simulink model "HANcoder_E407_DYS_MP"  (R2018b)
settings: Solver=FixedStepDiscrete  StartTime=0.0  StopTime=1  FixedStep=0.01  RelTol=1e-3
PreLoadFcn:
  | librarySetup
  | eval([bdroot,'_startup']) %Calling [modelName]_startup.m
values from neighbouring files (symbols this model uses):
  basic_cycle_duration_bc0 = TM_Reset_Board   + COMP_duration    (= 212)    [HANcoder_E407_DYS_MP_startup.m]
  basic_cycle_duration_bc1 = basic_cycle_duration_bc0    (= 212)    [HANcoder_E407_DYS_MP_startup.m]
  comm_delay_estimation1 = round(comm_delay_measured1*hardware_granularity/frequency_IRQ)    [HANcoder_E407_DYS_MP_startup.m]
  comm_delay_estimation2 = round(comm_delay_measured2*hardware_granularity/frequency_IRQ)    [HANcoder_E407_DYS_MP_startup.m]
  COMM_Phase1 = Simulink.Parameter    [HANcoder_E407_DYS_MP_startup.m]
  COMM_Phase2 = Simulink.Parameter    [HANcoder_E407_DYS_MP_startup.m]
  frequency_IRQ = 500    [HANcoder_E407_DYS_MP_startup.m]
  HantuneAngleSp = Simulink.Parameter    [HANcoder_E407_DYS_MP_startup.m]
  idle_time_init = basic_cycle_duration_bc0 + basic_cycle_duration_bc1    (= 424)    [HANcoder_E407_DYS_MP_startup.m]
  matrix_rows = 2    [HANcoder_E407_DYS_MP_startup.m]
  positionD = Simulink.Parameter    [HANcoder_E407_DYS_MP_startup.m]
  positionI = Simulink.Parameter    [HANcoder_E407_DYS_MP_startup.m]
  positionP = Simulink.Parameter    [HANcoder_E407_DYS_MP_startup.m]
undefined symbols (not defined in the file or in its folder): A1, CON2, CON4, D13, Dposition, Iposition, Pposition
libraries: HANcoder_STM32_Target x33, dspswit3 x16, simulink x2, simulink_extras x2, dspstat3 x1
(part 7 of 10)

== system HANcoder_E407_DYS_MP/HANcoder STM32 Target - E407-STM32 algorithm/4.TTA Can System/4.3 TTA System/4.3.3 Matrix Cycle Manager/4.3.3.1 Controller Matrix Cycle Truck Boards 1 2 and 3/4.3.3.1.2 controller basic cycle 0.2/Receive Truck 1 Board 1 Calc Steering Angle/Receive can message ==
  Can_ID : Inport
  Enable : EnablePort  ShowOutputPort=on
  CAN receive : Subsystem  Tag=HANcoder_TARGET_STM32_E407  AncestorBlock=HANcoder_STM32_Target/STM32-E407/CAN/CAN/CAN receive  mask(CAN receive){canBus=CAN 1, outputNumber=1, dataType=uint8, byteOrder=off, tsamp=-1}
      mask prompts: canBus "CAN channel"; outputNumber "Output ports"; dataType "Output datatype"; byteOrder "Byte order: Checked = MSB first, unchecked = LSB first."; tsamp "Sample time"
      mask help:
      | Function
      | ==========
      | Receive the newest message from the specified CAN channel.
      |
      | Parameters
      | ==========
      | CAN channel:             The CAN channel to send the message on.
      | Output ports:             The amount of output ports
      | Output datatype:       The datatype of the output ports
      | Byte order:                 Select MSB or LSB first
      | Sample time:              -1 or divisible by base sample time [seconds]
      |
      | Input
      | ==========
      | Port 1:                       CAN ID(uint32) in hexadecimal ie: hex2dec('0a')
      |
      | Output
      | ==========
      | Port 1:                       Checks for new message(int8)
      | Port 2..9                     Message data
      mask init:
      | sfcn_can_receive_mcb(canBus, outputNumber, dataType, byteOrder)
      settings: MoveFcn=drawLogos
      mask Help: web('sfcn_can_receive.html');
      mask TypeOptions canBus: CAN 1 | CAN 2
      mask TypeOptions dataType: int8 | uint8 | int16 | uint16 | int32 | uint32 | boolean
      mask Display:
      | fprintf('Receive on\nCAN %x', canBus);
      | port_label('output', 1, 'new');
      | port_label('input', 1, 'ID');patch([75 81 81],[8 14 2],[1 0 0]);patch([83 83 89],[14 2 8],[0 0 0.35]);
  CAN receive2 : Subsystem  Tag=HANcoder_TARGET_STM32_E407  AncestorBlock=HANcoder_STM32_Target/STM32-E407/CAN/CAN/CAN receive  mask(CAN receive){canBus=CAN 2, outputNumber=1, dataType=uint8, byteOrder=off, tsamp=-1}
      mask prompts: canBus "CAN channel"; outputNumber "Output ports"; dataType "Output datatype"; byteOrder "Byte order: Checked = MSB first, unchecked = LSB first."; tsamp "Sample time"
      mask help:
      | Function
      | ==========
      | Receive the newest message from the specified CAN channel.
      |
      | Parameters
      | ==========
      | CAN channel:             The CAN channel to send the message on.
      | Output ports:             The amount of output ports
      | Output datatype:       The datatype of the output ports
      | Byte order:                 Select MSB or LSB first
      | Sample time:              -1 or divisible by base sample time [seconds]
      |
      | Input
      | ==========
      | Port 1:                       CAN ID(uint32) in hexadecimal ie: hex2dec('0a')
      |
      | Output
      | ==========
      | Port 1:                       Checks for new message(int8)
      | Port 2..9                     Message data
      mask init:
      | sfcn_can_receive_mcb(canBus, outputNumber, dataType, byteOrder)
      settings: MoveFcn=drawLogos
      mask Help: web('sfcn_can_receive.html');
      mask TypeOptions canBus: CAN 1 | CAN 2
      mask TypeOptions dataType: int8 | uint8 | int16 | uint16 | int32 | uint32 | boolean
      mask Display:
      | fprintf('Receive on\nCAN %x', canBus);
      | port_label('output', 1, 'new');
      | port_label('input', 1, 'ID');patch([75 81 81],[8 14 2],[1 0 0]);patch([83 83 89],[14 2 8],[0 0 0.35]);
  Can1Port1 : Outport
  Can1Receive : Outport  Port=2
  Can2Port2 : Outport  Port=3
  Can2Receive : Outport  Port=4
  wires:
  CAN receive/2(Out2) -> Can1Port1/1
  CAN receive/1(Out1) -> Can1Receive/1
  Can_ID/1 -> CAN receive2/1(In1), CAN receive/1(In1)
  CAN receive2/1(Out1) -> Can2Receive/1
  CAN receive2/2(Out2) -> Can2Port2/1

== system HANcoder_E407_DYS_MP/HANcoder STM32 Target - E407-STM32 algorithm/4.TTA Can System/4.3 TTA System/4.3.3 Matrix Cycle Manager/4.3.3.1 Controller Matrix Cycle Truck Boards 1 2 and 3/4.3.3.1.2 controller basic cycle 0.2/Receive Truck 1 Board 1 Calc Steering Angle1/Desync calculation ==
  New_msg_CAN1 : Inport
  Can1_Msg : Inport  Port=2
  Can2_Msg : Inport  Port=3
  Enable : EnablePort  ShowOutputPort=on
  Switch1 : Switch  Priority=22  Criteria=u2 > Threshold
  Vote : Outport
  wires:
  New_msg_CAN1/1 -> Switch1/2
  Can1_Msg/1 -> Switch1/1
  Can2_Msg/1 -> Switch1/3
  Switch1/1 -> Vote/1

== system HANcoder_E407_DYS_MP/HANcoder STM32 Target - E407-STM32 algorithm/4.TTA Can System/4.3 TTA System/4.3.3 Matrix Cycle Manager/4.3.3.1 Controller Matrix Cycle Truck Boards 1 2 and 3/4.3.3.1.2 controller basic cycle 0.2/Receive Truck 1 Board 1 Calc Steering Angle1/Receive can message ==
  Can_ID : Inport
  Enable : EnablePort  ShowOutputPort=on
  CAN receive : Subsystem  Tag=HANcoder_TARGET_STM32_E407  AncestorBlock=HANcoder_STM32_Target/STM32-E407/CAN/CAN/CAN receive  mask(CAN receive){canBus=CAN 1, outputNumber=1, dataType=uint8, byteOrder=off, tsamp=-1}
      mask prompts: canBus "CAN channel"; outputNumber "Output ports"; dataType "Output datatype"; byteOrder "Byte order: Checked = MSB first, unchecked = LSB first."; tsamp "Sample time"
      mask help:
      | Function
      | ==========
      | Receive the newest message from the specified CAN channel.
      |
      | Parameters
      | ==========
      | CAN channel:             The CAN channel to send the message on.
      | Output ports:             The amount of output ports
      | Output datatype:       The datatype of the output ports
      | Byte order:                 Select MSB or LSB first
      | Sample time:              -1 or divisible by base sample time [seconds]
      |
      | Input
      | ==========
      | Port 1:                       CAN ID(uint32) in hexadecimal ie: hex2dec('0a')
      |
      | Output
      | ==========
      | Port 1:                       Checks for new message(int8)
      | Port 2..9                     Message data
      mask init:
      | sfcn_can_receive_mcb(canBus, outputNumber, dataType, byteOrder)
      settings: MoveFcn=drawLogos
      mask Help: web('sfcn_can_receive.html');
      mask TypeOptions canBus: CAN 1 | CAN 2
      mask TypeOptions dataType: int8 | uint8 | int16 | uint16 | int32 | uint32 | boolean
      mask Display:
      | fprintf('Receive on\nCAN %x', canBus);
      | port_label('output', 1, 'new');
      | port_label('input', 1, 'ID');patch([75 81 81],[8 14 2],[1 0 0]);patch([83 83 89],[14 2 8],[0 0 0.35]);
  CAN receive2 : Subsystem  Tag=HANcoder_TARGET_STM32_E407  AncestorBlock=HANcoder_STM32_Target/STM32-E407/CAN/CAN/CAN receive  mask(CAN receive){canBus=CAN 2, outputNumber=1, dataType=uint8, byteOrder=off, tsamp=-1}
      mask prompts: canBus "CAN channel"; outputNumber "Output ports"; dataType "Output datatype"; byteOrder "Byte order: Checked = MSB first, unchecked = LSB first."; tsamp "Sample time"
      mask help:
      | Function
      | ==========
      | Receive the newest message from the specified CAN channel.
      |
      | Parameters
      | ==========
      | CAN channel:             The CAN channel to send the message on.
      | Output ports:             The amount of output ports
      | Output datatype:       The datatype of the output ports
      | Byte order:                 Select MSB or LSB first
      | Sample time:              -1 or divisible by base sample time [seconds]
      |
      | Input
      | ==========
      | Port 1:                       CAN ID(uint32) in hexadecimal ie: hex2dec('0a')
      |
      | Output
      | ==========
      | Port 1:                       Checks for new message(int8)
      | Port 2..9                     Message data
      mask init:
      | sfcn_can_receive_mcb(canBus, outputNumber, dataType, byteOrder)
      settings: MoveFcn=drawLogos
      mask Help: web('sfcn_can_receive.html');
      mask TypeOptions canBus: CAN 1 | CAN 2
      mask TypeOptions dataType: int8 | uint8 | int16 | uint16 | int32 | uint32 | boolean
      mask Display:
      | fprintf('Receive on\nCAN %x', canBus);
      | port_label('output', 1, 'new');
      | port_label('input', 1, 'ID');patch([75 81 81],[8 14 2],[1 0 0]);patch([83 83 89],[14 2 8],[0 0 0.35]);
  Can1Port1 : Outport
  Can1Receive : Outport  Port=2
  Can2Port2 : Outport  Port=3
  Can2Receive : Outport  Port=4
  wires:
  CAN receive/2(Out2) -> Can1Port1/1
  CAN receive/1(Out1) -> Can1Receive/1
  Can_ID/1 -> CAN receive2/1(In1), CAN receive/1(In1)
  CAN receive2/1(Out1) -> Can2Receive/1
  CAN receive2/2(Out2) -> Can2Port2/1

== system HANcoder_E407_DYS_MP/HANcoder STM32 Target - E407-STM32 algorithm/4.TTA Can System/4.3 TTA System/4.3.3 Matrix Cycle Manager/4.3.3.1 Controller Matrix Cycle Truck Boards 1 2 and 3/4.3.3.1.2 controller basic cycle 0.2/Receive Truck 1 Board 1 Calc Steering Angle2/Desync calculation ==
  New_msg_CAN1 : Inport
  Can1_Msg : Inport  Port=2
  Can2_Msg : Inport  Port=3
  Enable : EnablePort  ShowOutputPort=on
  Switch1 : Switch  Priority=22  Criteria=u2 > Threshold
  Vote : Outport
  wires:
  New_msg_CAN1/1 -> Switch1/2
  Can1_Msg/1 -> Switch1/1
  Can2_Msg/1 -> Switch1/3
  Switch1/1 -> Vote/1

== system HANcoder_E407_DYS_MP/HANcoder STM32 Target - E407-STM32 algorithm/4.TTA Can System/4.3 TTA System/4.3.3 Matrix Cycle Manager/4.3.3.1 Controller Matrix Cycle Truck Boards 1 2 and 3/4.3.3.1.2 controller basic cycle 0.2/Receive Truck 1 Board 1 Calc Steering Angle2/Receive can message ==
  Can_ID : Inport
  Enable : EnablePort  ShowOutputPort=on
  CAN receive : Subsystem  Tag=HANcoder_TARGET_STM32_E407  AncestorBlock=HANcoder_STM32_Target/STM32-E407/CAN/CAN/CAN receive  mask(CAN receive){canBus=CAN 1, outputNumber=1, dataType=uint8, byteOrder=off, tsamp=-1}
      mask prompts: canBus "CAN channel"; outputNumber "Output ports"; dataType "Output datatype"; byteOrder "Byte order: Checked = MSB first, unchecked = LSB first."; tsamp "Sample time"
      mask help:
      | Function
      | ==========
      | Receive the newest message from the specified CAN channel.
      |
      | Parameters
      | ==========
      | CAN channel:             The CAN channel to send the message on.
      | Output ports:             The amount of output ports
      | Output datatype:       The datatype of the output ports
      | Byte order:                 Select MSB or LSB first
      | Sample time:              -1 or divisible by base sample time [seconds]
      |
      | Input
      | ==========
      | Port 1:                       CAN ID(uint32) in hexadecimal ie: hex2dec('0a')
      |
      | Output
      | ==========
      | Port 1:                       Checks for new message(int8)
      | Port 2..9                     Message data
      mask init:
      | sfcn_can_receive_mcb(canBus, outputNumber, dataType, byteOrder)
      settings: MoveFcn=drawLogos
      mask Help: web('sfcn_can_receive.html');
      mask TypeOptions canBus: CAN 1 | CAN 2
      mask TypeOptions dataType: int8 | uint8 | int16 | uint16 | int32 | uint32 | boolean
      mask Display:
      | fprintf('Receive on\nCAN %x', canBus);
      | port_label('output', 1, 'new');
      | port_label('input', 1, 'ID');patch([75 81 81],[8 14 2],[1 0 0]);patch([83 83 89],[14 2 8],[0 0 0.35]);
  CAN receive2 : Subsystem  Tag=HANcoder_TARGET_STM32_E407  AncestorBlock=HANcoder_STM32_Target/STM32-E407/CAN/CAN/CAN receive  mask(CAN receive){canBus=CAN 2, outputNumber=1, dataType=uint8, byteOrder=off, tsamp=-1}
      mask prompts: canBus "CAN channel"; outputNumber "Output ports"; dataType "Output datatype"; byteOrder "Byte order: Checked = MSB first, unchecked = LSB first."; tsamp "Sample time"
      mask help:
      | Function
      | ==========
      | Receive the newest message from the specified CAN channel.
      |
      | Parameters
      | ==========
      | CAN channel:             The CAN channel to send the message on.
      | Output ports:             The amount of output ports
      | Output datatype:       The datatype of the output ports
      | Byte order:                 Select MSB or LSB first
      | Sample time:              -1 or divisible by base sample time [seconds]
      |
      | Input
      | ==========
      | Port 1:                       CAN ID(uint32) in hexadecimal ie: hex2dec('0a')
      |
      | Output
      | ==========
      | Port 1:                       Checks for new message(int8)
      | Port 2..9                     Message data
      mask init:
      | sfcn_can_receive_mcb(canBus, outputNumber, dataType, byteOrder)
      settings: MoveFcn=drawLogos
      mask Help: web('sfcn_can_receive.html');
      mask TypeOptions canBus: CAN 1 | CAN 2
      mask TypeOptions dataType: int8 | uint8 | int16 | uint16 | int32 | uint32 | boolean
      mask Display:
      | fprintf('Receive on\nCAN %x', canBus);
      | port_label('output', 1, 'new');
      | port_label('input', 1, 'ID');patch([75 81 81],[8 14 2],[1 0 0]);patch([83 83 89],[14 2 8],[0 0 0.35]);
  Can1Port1 : Outport
  Can1Receive : Outport  Port=2
  Can2Port2 : Outport  Port=3
  Can2Receive : Outport  Port=4
  wires:
  CAN receive/2(Out2) -> Can1Port1/1
  CAN receive/1(Out1) -> Can1Receive/1
  Can_ID/1 -> CAN receive2/1(In1), CAN receive/1(In1)
  CAN receive2/1(Out1) -> Can2Receive/1
  CAN receive2/2(Out2) -> Can2Port2/1

== system HANcoder_E407_DYS_MP/HANcoder STM32 Target - E407-STM32 algorithm/4.TTA Can System/4.3 TTA System/4.3.3 Matrix Cycle Manager/4.3.3.1 Controller Matrix Cycle Truck Boards 1 2 and 3/4.3.3.1.2 controller basic cycle 0.2/Receive Truck 1 Board 1 Calc Steering Angle3/Desync calculation ==
  New_msg_CAN1 : Inport
  Can1_Msg : Inport  Port=2
  Can2_Msg : Inport  Port=3
  Enable : EnablePort  ShowOutputPort=on
  Switch1 : Switch  Priority=22  Criteria=u2 > Threshold
  Vote : Outport
  wires:
  New_msg_CAN1/1 -> Switch1/2
  Can1_Msg/1 -> Switch1/1
  Can2_Msg/1 -> Switch1/3
  Switch1/1 -> Vote/1

== system HANcoder_E407_DYS_MP/HANcoder STM32 Target - E407-STM32 algorithm/4.TTA Can System/4.3 TTA System/4.3.3 Matrix Cycle Manager/4.3.3.1 Controller Matrix Cycle Truck Boards 1 2 and 3/4.3.3.1.2 controller basic cycle 0.2/Receive Truck 1 Board 1 Calc Steering Angle3/Receive can message ==
  Can_ID : Inport
  Enable : EnablePort  ShowOutputPort=on
  CAN receive : Subsystem  Tag=HANcoder_TARGET_STM32_E407  AncestorBlock=HANcoder_STM32_Target/STM32-E407/CAN/CAN/CAN receive  mask(CAN receive){canBus=CAN 1, outputNumber=1, dataType=uint8, byteOrder=off, tsamp=-1}
      mask prompts: canBus "CAN channel"; outputNumber "Output ports"; dataType "Output datatype"; byteOrder "Byte order: Checked = MSB first, unchecked = LSB first."; tsamp "Sample time"
      mask help:
      | Function
      | ==========
      | Receive the newest message from the specified CAN channel.
      |
      | Parameters
      | ==========
      | CAN channel:             The CAN channel to send the message on.
      | Output ports:             The amount of output ports
      | Output datatype:       The datatype of the output ports
      | Byte order:                 Select MSB or LSB first
      | Sample time:              -1 or divisible by base sample time [seconds]
      |
      | Input
      | ==========
      | Port 1:                       CAN ID(uint32) in hexadecimal ie: hex2dec('0a')
      |
      | Output
      | ==========
      | Port 1:                       Checks for new message(int8)
      | Port 2..9                     Message data
      mask init:
      | sfcn_can_receive_mcb(canBus, outputNumber, dataType, byteOrder)
      settings: MoveFcn=drawLogos
      mask Help: web('sfcn_can_receive.html');
      mask TypeOptions canBus: CAN 1 | CAN 2
      mask TypeOptions dataType: int8 | uint8 | int16 | uint16 | int32 | uint32 | boolean
      mask Display:
      | fprintf('Receive on\nCAN %x', canBus);
      | port_label('output', 1, 'new');
      | port_label('input', 1, 'ID');patch([75 81 81],[8 14 2],[1 0 0]);patch([83 83 89],[14 2 8],[0 0 0.35]);
  CAN receive2 : Subsystem  Tag=HANcoder_TARGET_STM32_E407  AncestorBlock=HANcoder_STM32_Target/STM32-E407/CAN/CAN/CAN receive  mask(CAN receive){canBus=CAN 2, outputNumber=1, dataType=uint8, byteOrder=off, tsamp=-1}
      mask prompts: canBus "CAN channel"; outputNumber "Output ports"; dataType "Output datatype"; byteOrder "Byte order: Checked = MSB first, unchecked = LSB first."; tsamp "Sample time"
      mask help:
      | Function
      | ==========
      | Receive the newest message from the specified CAN channel.
      |
      | Parameters
      | ==========
      | CAN channel:             The CAN channel to send the message on.
      | Output ports:             The amount of output ports
      | Output datatype:       The datatype of the output ports
      | Byte order:                 Select MSB or LSB first
      | Sample time:              -1 or divisible by base sample time [seconds]
      |
      | Input
      | ==========
      | Port 1:                       CAN ID(uint32) in hexadecimal ie: hex2dec('0a')
      |
      | Output
      | ==========
      | Port 1:                       Checks for new message(int8)
      | Port 2..9                     Message data
      mask init:
      | sfcn_can_receive_mcb(canBus, outputNumber, dataType, byteOrder)
      settings: MoveFcn=drawLogos
      mask Help: web('sfcn_can_receive.html');
      mask TypeOptions canBus: CAN 1 | CAN 2
      mask TypeOptions dataType: int8 | uint8 | int16 | uint16 | int32 | uint32 | boolean
      mask Display:
      | fprintf('Receive on\nCAN %x', canBus);
      | port_label('output', 1, 'new');
      | port_label('input', 1, 'ID');patch([75 81 81],[8 14 2],[1 0 0]);patch([83 83 89],[14 2 8],[0 0 0.35]);
  Can1Port1 : Outport
  Can1Receive : Outport  Port=2
  Can2Port2 : Outport  Port=3
  Can2Receive : Outport  Port=4
  wires:
  CAN receive/2(Out2) -> Can1Port1/1
  CAN receive/1(Out1) -> Can1Receive/1
  Can_ID/1 -> CAN receive2/1(In1), CAN receive/1(In1)
  CAN receive2/1(Out1) -> Can2Receive/1
  CAN receive2/2(Out2) -> Can2Port2/1

== system HANcoder_E407_DYS_MP/HANcoder STM32 Target - E407-STM32 algorithm/4.TTA Can System/4.3 TTA System/4.3.3 Matrix Cycle Manager/4.3.3.1 Controller Matrix Cycle Truck Boards 1 2 and 3/4.3.3.1.2 controller basic cycle 0.2/Receive Truck 2 Board 2 Calc Steering Angle/Desync calculation ==
  New_msg_CAN1 : Inport
  Can1_Msg : Inport  Port=2
  Can2_Msg : Inport  Port=3
  Enable : EnablePort  ShowOutputPort=on
  Switch1 : Switch  Priority=22  Criteria=u2 > Threshold
  Vote : Outport
  wires:
  New_msg_CAN1/1 -> Switch1/2
  Can1_Msg/1 -> Switch1/1
  Can2_Msg/1 -> Switch1/3
  Switch1/1 -> Vote/1

== system HANcoder_E407_DYS_MP/HANcoder STM32 Target - E407-STM32 algorithm/4.TTA Can System/4.3 TTA System/4.3.3 Matrix Cycle Manager/4.3.3.1 Controller Matrix Cycle Truck Boards 1 2 and 3/4.3.3.1.2 controller basic cycle 0.2/Receive Truck 2 Board 2 Calc Steering Angle/Receive can message ==
  Can_ID : Inport
  Enable : EnablePort  ShowOutputPort=on
  CAN receive : Subsystem  Tag=HANcoder_TARGET_STM32_E407  AncestorBlock=HANcoder_STM32_Target/STM32-E407/CAN/CAN/CAN receive  mask(CAN receive){canBus=CAN 1, outputNumber=1, dataType=uint8, byteOrder=off, tsamp=-1}
      mask prompts: canBus "CAN channel"; outputNumber "Output ports"; dataType "Output datatype"; byteOrder "Byte order: Checked = MSB first, unchecked = LSB first."; tsamp "Sample time"
      mask help:
      | Function
      | ==========
      | Receive the newest message from the specified CAN channel.
      |
      | Parameters
      | ==========
      | CAN channel:             The CAN channel to send the message on.
      | Output ports:             The amount of output ports
      | Output datatype:       The datatype of the output ports
      | Byte order:                 Select MSB or LSB first
      | Sample time:              -1 or divisible by base sample time [seconds]
      |
      | Input
      | ==========
      | Port 1:                       CAN ID(uint32) in hexadecimal ie: hex2dec('0a')
      |
      | Output
      | ==========
      | Port 1:                       Checks for new message(int8)
      | Port 2..9                     Message data
      mask init:
      | sfcn_can_receive_mcb(canBus, outputNumber, dataType, byteOrder)
      settings: MoveFcn=drawLogos
      mask Help: web('sfcn_can_receive.html');
      mask TypeOptions canBus: CAN 1 | CAN 2
      mask TypeOptions dataType: int8 | uint8 | int16 | uint16 | int32 | uint32 | boolean
      mask Display:
      | fprintf('Receive on\nCAN %x', canBus);
      | port_label('output', 1, 'new');
      | port_label('input', 1, 'ID');patch([75 81 81],[8 14 2],[1 0 0]);patch([83 83 89],[14 2 8],[0 0 0.35]);
  CAN receive2 : Subsystem  Tag=HANcoder_TARGET_STM32_E407  AncestorBlock=HANcoder_STM32_Target/STM32-E407/CAN/CAN/CAN receive  mask(CAN receive){canBus=CAN 2, outputNumber=1, dataType=uint8, byteOrder=off, tsamp=-1}
      mask prompts: canBus "CAN channel"; outputNumber "Output ports"; dataType "Output datatype"; byteOrder "Byte order: Checked = MSB first, unchecked = LSB first."; tsamp "Sample time"
      mask help:
      | Function
      | ==========
      | Receive the newest message from the specified CAN channel.
      |
      | Parameters
      | ==========
      | CAN channel:             The CAN channel to send the message on.
      | Output ports:             The amount of output ports
      | Output datatype:       The datatype of the output ports
      | Byte order:                 Select MSB or LSB first
      | Sample time:              -1 or divisible by base sample time [seconds]
      |
      | Input
      | ==========
      | Port 1:                       CAN ID(uint32) in hexadecimal ie: hex2dec('0a')
      |
      | Output
      | ==========
      | Port 1:                       Checks for new message(int8)
      | Port 2..9                     Message data
      mask init:
      | sfcn_can_receive_mcb(canBus, outputNumber, dataType, byteOrder)
      settings: MoveFcn=drawLogos
      mask Help: web('sfcn_can_receive.html');
      mask TypeOptions canBus: CAN 1 | CAN 2
      mask TypeOptions dataType: int8 | uint8 | int16 | uint16 | int32 | uint32 | boolean
      mask Display:
      | fprintf('Receive on\nCAN %x', canBus);
      | port_label('output', 1, 'new');
      | port_label('input', 1, 'ID');patch([75 81 81],[8 14 2],[1 0 0]);patch([83 83 89],[14 2 8],[0 0 0.35]);
  Can1Port1 : Outport
  Can1Receive : Outport  Port=2
  Can2Port2 : Outport  Port=3
  Can2Receive : Outport  Port=4
  wires:
  CAN receive/2(Out2) -> Can1Port1/1
  CAN receive/1(Out1) -> Can1Receive/1
  Can_ID/1 -> CAN receive2/1(In1), CAN receive/1(In1)
  CAN receive2/1(Out1) -> Can2Receive/1
  CAN receive2/2(Out2) -> Can2Port2/1

== system HANcoder_E407_DYS_MP/HANcoder STM32 Target - E407-STM32 algorithm/4.TTA Can System/4.3 TTA System/4.3.3 Matrix Cycle Manager/4.3.3.1 Controller Matrix Cycle Truck Boards 1 2 and 3/4.3.3.1.2 controller basic cycle 0.2/Receive Truck 3 Board 3 Calc Steering Angle/Desync calculation ==
  New_msg_CAN1 : Inport
  Can1_Msg : Inport  Port=2
  Can2_Msg : Inport  Port=3
  Enable : EnablePort  ShowOutputPort=on
  Switch1 : Switch  Priority=22  Criteria=u2 > Threshold
  Vote : Outport
  wires:
  New_msg_CAN1/1 -> Switch1/2
  Can1_Msg/1 -> Switch1/1
  Can2_Msg/1 -> Switch1/3
  Switch1/1 -> Vote/1

== system HANcoder_E407_DYS_MP/HANcoder STM32 Target - E407-STM32 algorithm/4.TTA Can System/4.3 TTA System/4.3.3 Matrix Cycle Manager/4.3.3.1 Controller Matrix Cycle Truck Boards 1 2 and 3/4.3.3.1.2 controller basic cycle 0.2/Receive Truck 3 Board 3 Calc Steering Angle/Receive can message ==
  Can_ID : Inport
  Enable : EnablePort  ShowOutputPort=on
  CAN receive : Subsystem  Tag=HANcoder_TARGET_STM32_E407  AncestorBlock=HANcoder_STM32_Target/STM32-E407/CAN/CAN/CAN receive  mask(CAN receive){canBus=CAN 1, outputNumber=1, dataType=uint8, byteOrder=off, tsamp=-1}
      mask prompts: canBus "CAN channel"; outputNumber "Output ports"; dataType "Output datatype"; byteOrder "Byte order: Checked = MSB first, unchecked = LSB first."; tsamp "Sample time"
      mask help:
      | Function
      | ==========
      | Receive the newest message from the specified CAN channel.
      |
      | Parameters
      | ==========
      | CAN channel:             The CAN channel to send the message on.
      | Output ports:             The amount of output ports
      | Output datatype:       The datatype of the output ports
      | Byte order:                 Select MSB or LSB first
      | Sample time:              -1 or divisible by base sample time [seconds]
      |
      | Input
      | ==========
      | Port 1:                       CAN ID(uint32) in hexadecimal ie: hex2dec('0a')
      |
      | Output
      | ==========
      | Port 1:                       Checks for new message(int8)
      | Port 2..9                     Message data
      mask init:
      | sfcn_can_receive_mcb(canBus, outputNumber, dataType, byteOrder)
      settings: MoveFcn=drawLogos
      mask Help: web('sfcn_can_receive.html');
      mask TypeOptions canBus: CAN 1 | CAN 2
      mask TypeOptions dataType: int8 | uint8 | int16 | uint16 | int32 | uint32 | boolean
      mask Display:
      | fprintf('Receive on\nCAN %x', canBus);
      | port_label('output', 1, 'new');
      | port_label('input', 1, 'ID');patch([75 81 81],[8 14 2],[1 0 0]);patch([83 83 89],[14 2 8],[0 0 0.35]);
  CAN receive2 : Subsystem  Tag=HANcoder_TARGET_STM32_E407  AncestorBlock=HANcoder_STM32_Target/STM32-E407/CAN/CAN/CAN receive  mask(CAN receive){canBus=CAN 2, outputNumber=1, dataType=uint8, byteOrder=off, tsamp=-1}
      mask prompts: canBus "CAN channel"; outputNumber "Output ports"; dataType "Output datatype"; byteOrder "Byte order: Checked = MSB first, unchecked = LSB first."; tsamp "Sample time"
      mask help:
      | Function
      | ==========
      | Receive the newest message from the specified CAN channel.
      |
      | Parameters
      | ==========
      | CAN channel:             The CAN channel to send the message on.
      | Output ports:             The amount of output ports
      | Output datatype:       The datatype of the output ports
      | Byte order:                 Select MSB or LSB first
      | Sample time:              -1 or divisible by base sample time [seconds]
      |
      | Input
      | ==========
      | Port 1:                       CAN ID(uint32) in hexadecimal ie: hex2dec('0a')
      |
      | Output
      | ==========
      | Port 1:                       Checks for new message(int8)
      | Port 2..9                     Message data
      mask init:
      | sfcn_can_receive_mcb(canBus, outputNumber, dataType, byteOrder)
      settings: MoveFcn=drawLogos
      mask Help: web('sfcn_can_receive.html');
      mask TypeOptions canBus: CAN 1 | CAN 2
      mask TypeOptions dataType: int8 | uint8 | int16 | uint16 | int32 | uint32 | boolean
      mask Display:
      | fprintf('Receive on\nCAN %x', canBus);
      | port_label('output', 1, 'new');
      | port_label('input', 1, 'ID');patch([75 81 81],[8 14 2],[1 0 0]);patch([83 83 89],[14 2 8],[0 0 0.35]);
  Can1Port1 : Outport
  Can1Receive : Outport  Port=2
  Can2Port2 : Outport  Port=3
  Can2Receive : Outport  Port=4
  wires:
  CAN receive/2(Out2) -> Can1Port1/1
  CAN receive/1(Out1) -> Can1Receive/1
  Can_ID/1 -> CAN receive2/1(In1), CAN receive/1(In1)
  CAN receive2/1(Out1) -> Can2Receive/1
  CAN receive2/2(Out2) -> Can2Port2/1

== system HANcoder_E407_DYS_MP/HANcoder STM32 Target - E407-STM32 algorithm/4.TTA Can System/4.3 TTA System/4.3.3 Matrix Cycle Manager/4.3.3.1 Controller Matrix Cycle Truck Boards 1 2 and 3/4.3.3.1.2 controller basic cycle 0.2/Send can message/CAN send ==
  In1 : Inport
  In2 : Inport  Port=2
  Gnd{3..9} (7 alike) : Ground
  S-Function : M-S-Function  FunctionName=sfcn_can_send  Parameters=tsamp, canBus, frameType, inputNumber, dataType, byteOrder
  wires:
  In1/1 -> S-Function/1
  In2/1 -> S-Function/2
  Gnd3/1 -> S-Function/3
  Gnd4/1 -> S-Function/4
  Gnd5/1 -> S-Function/5
  Gnd6/1 -> S-Function/6
  Gnd7/1 -> S-Function/7
  Gnd8/1 -> S-Function/8
  Gnd9/1 -> S-Function/9

== system HANcoder_E407_DYS_MP/HANcoder STM32 Target - E407-STM32 algorithm/4.TTA Can System/4.3 TTA System/4.3.3 Matrix Cycle Manager/4.3.3.1 Controller Matrix Cycle Truck Boards 1 2 and 3/4.3.3.1.2 controller basic cycle 0.2/Send can message/CAN send1 ==
  In1 : Inport
  In2 : Inport  Port=2
  Gnd{3..9} (7 alike) : Ground
  S-Function : M-S-Function  FunctionName=sfcn_can_send  Parameters=tsamp, canBus, frameType, inputNumber, dataType, byteOrder
  wires:
  In1/1 -> S-Function/1
  In2/1 -> S-Function/2
  Gnd3/1 -> S-Function/3
  Gnd4/1 -> S-Function/4
  Gnd5/1 -> S-Function/5
  Gnd6/1 -> S-Function/6
  Gnd7/1 -> S-Function/7
  Gnd8/1 -> S-Function/8
  Gnd9/1 -> S-Function/9

== system HANcoder_E407_DYS_MP/HANcoder STM32 Target - E407-STM32 algorithm/4.TTA Can System/4.3 TTA System/4.3.3 Matrix Cycle Manager/4.3.3.1 Controller Matrix Cycle Truck Boards 1 2 and 3/4.3.3.1.2 controller basic cycle 0.2/Send can message1/CAN send ==
  In1 : Inport
  In2 : Inport  Port=2
  Gnd{3..9} (7 alike) : Ground
  S-Function : M-S-Function  FunctionName=sfcn_can_send  Parameters=tsamp, canBus, frameType, inputNumber, dataType, byteOrder
  wires:
  In1/1 -> S-Function/1
  In2/1 -> S-Function/2
  Gnd3/1 -> S-Function/3
  Gnd4/1 -> S-Function/4
  Gnd5/1 -> S-Function/5
  Gnd6/1 -> S-Function/6
  Gnd7/1 -> S-Function/7
  Gnd8/1 -> S-Function/8
  Gnd9/1 -> S-Function/9

== system HANcoder_E407_DYS_MP/HANcoder STM32 Target - E407-STM32 algorithm/4.TTA Can System/4.3 TTA System/4.3.3 Matrix Cycle Manager/4.3.3.1 Controller Matrix Cycle Truck Boards 1 2 and 3/4.3.3.1.2 controller basic cycle 0.2/Send can message1/CAN send1 ==
  In1 : Inport
  In2 : Inport  Port=2
  Gnd{3..9} (7 alike) : Ground
  S-Function : M-S-Function  FunctionName=sfcn_can_send  Parameters=tsamp, canBus, frameType, inputNumber, dataType, byteOrder
  wires:
  In1/1 -> S-Function/1
  In2/1 -> S-Function/2
  Gnd3/1 -> S-Function/3
  Gnd4/1 -> S-Function/4
  Gnd5/1 -> S-Function/5
  Gnd6/1 -> S-Function/6
  Gnd7/1 -> S-Function/7
  Gnd8/1 -> S-Function/8
  Gnd9/1 -> S-Function/9

== system HANcoder_E407_DYS_MP/HANcoder STM32 Target - E407-STM32 algorithm/4.TTA Can System/4.3 TTA System/4.3.3 Matrix Cycle Manager/4.3.3.1 Controller Matrix Cycle Truck Boards 1 2 and 3/4.3.3.1.2 controller basic cycle 0.2/Send can message2/CAN send ==
  In1 : Inport
  In2 : Inport  Port=2
  Gnd{3..9} (7 alike) : Ground
  S-Function : M-S-Function  FunctionName=sfcn_can_send  Parameters=tsamp, canBus, frameType, inputNumber, dataType, byteOrder
  wires:
  In1/1 -> S-Function/1
  In2/1 -> S-Function/2
  Gnd3/1 -> S-Function/3
  Gnd4/1 -> S-Function/4
  Gnd5/1 -> S-Function/5
  Gnd6/1 -> S-Function/6
  Gnd7/1 -> S-Function/7
  Gnd8/1 -> S-Function/8
  Gnd9/1 -> S-Function/9

== system HANcoder_E407_DYS_MP/HANcoder STM32 Target - E407-STM32 algorithm/4.TTA Can System/4.3 TTA System/4.3.3 Matrix Cycle Manager/4.3.3.1 Controller Matrix Cycle Truck Boards 1 2 and 3/4.3.3.1.2 controller basic cycle 0.2/Send can message2/CAN send1 ==
  In1 : Inport
  In2 : Inport  Port=2
  Gnd{3..9} (7 alike) : Ground
  S-Function : M-S-Function  FunctionName=sfcn_can_send  Parameters=tsamp, canBus, frameType, inputNumber, dataType, byteOrder
  wires:
  In1/1 -> S-Function/1
  In2/1 -> S-Function/2
  Gnd3/1 -> S-Function/3
  Gnd4/1 -> S-Function/4
  Gnd5/1 -> S-Function/5
  Gnd6/1 -> S-Function/6
  Gnd7/1 -> S-Function/7
  Gnd8/1 -> S-Function/8
  Gnd9/1 -> S-Function/9

== system HANcoder_E407_DYS_MP/HANcoder STM32 Target - E407-STM32 algorithm/4.TTA Can System/4.3 TTA System/4.3.3 Matrix Cycle Manager/4.3.3.1 Controller Matrix Cycle Truck Boards 1 2 and 3/4.3.3.1.2 controller basic cycle 0.2/Send can message3/CAN send ==
  In1 : Inport
  In2 : Inport  Port=2
  Gnd{3..9} (7 alike) : Ground
  S-Function : M-S-Function  FunctionName=sfcn_can_send  Parameters=tsamp, canBus, frameType, inputNumber, dataType, byteOrder
  wires:
  In1/1 -> S-Function/1
  In2/1 -> S-Function/2
  Gnd3/1 -> S-Function/3
  Gnd4/1 -> S-Function/4
  Gnd5/1 -> S-Function/5
  Gnd6/1 -> S-Function/6
  Gnd7/1 -> S-Function/7
  Gnd8/1 -> S-Function/8
  Gnd9/1 -> S-Function/9

== system HANcoder_E407_DYS_MP/HANcoder STM32 Target - E407-STM32 algorithm/4.TTA Can System/4.3 TTA System/4.3.3 Matrix Cycle Manager/4.3.3.1 Controller Matrix Cycle Truck Boards 1 2 and 3/4.3.3.1.2 controller basic cycle 0.2/Send can message3/CAN send1 ==
  In1 : Inport
  In2 : Inport  Port=2
  Gnd{3..9} (7 alike) : Ground
  S-Function : M-S-Function  FunctionName=sfcn_can_send  Parameters=tsamp, canBus, frameType, inputNumber, dataType, byteOrder
  wires:
  In1/1 -> S-Function/1
  In2/1 -> S-Function/2
  Gnd3/1 -> S-Function/3
  Gnd4/1 -> S-Function/4
  Gnd5/1 -> S-Function/5
  Gnd6/1 -> S-Function/6
  Gnd7/1 -> S-Function/7
  Gnd8/1 -> S-Function/8
  Gnd9/1 -> S-Function/9

== system HANcoder_E407_DYS_MP/HANcoder STM32 Target - E407-STM32 algorithm/4.TTA Can System/4.3 TTA System/4.3.3 Matrix Cycle Manager/4.3.3.1 Controller Matrix Cycle Truck Boards 1 2 and 3/4.3.3.1.2 controller basic cycle 0.2/Send can message4/CAN send ==
  In1 : Inport
  In2 : Inport  Port=2
  Gnd{3..9} (7 alike) : Ground
  S-Function : M-S-Function  FunctionName=sfcn_can_send  Parameters=tsamp, canBus, frameType, inputNumber, dataType, byteOrder
  wires:
  In1/1 -> S-Function/1
  In2/1 -> S-Function/2
  Gnd3/1 -> S-Function/3
  Gnd4/1 -> S-Function/4
  Gnd5/1 -> S-Function/5
  Gnd6/1 -> S-Function/6
  Gnd7/1 -> S-Function/7
  Gnd8/1 -> S-Function/8
  Gnd9/1 -> S-Function/9

== system HANcoder_E407_DYS_MP/HANcoder STM32 Target - E407-STM32 algorithm/4.TTA Can System/4.3 TTA System/4.3.3 Matrix Cycle Manager/4.3.3.1 Controller Matrix Cycle Truck Boards 1 2 and 3/4.3.3.1.2 controller basic cycle 0.2/Send can message4/CAN send1 ==
  In1 : Inport
  In2 : Inport  Port=2
  Gnd{3..9} (7 alike) : Ground
  S-Function : M-S-Function  FunctionName=sfcn_can_send  Parameters=tsamp, canBus, frameType, inputNumber, dataType, byteOrder
  wires:
  In1/1 -> S-Function/1
  In2/1 -> S-Function/2
  Gnd3/1 -> S-Function/3
  Gnd4/1 -> S-Function/4
  Gnd5/1 -> S-Function/5
  Gnd6/1 -> S-Function/6
  Gnd7/1 -> S-Function/7
  Gnd8/1 -> S-Function/8
  Gnd9/1 -> S-Function/9

== system HANcoder_E407_DYS_MP/HANcoder STM32 Target - E407-STM32 algorithm/4.TTA Can System/4.3 TTA System/4.3.3 Matrix Cycle Manager/4.3.3.1 Controller Matrix Cycle Truck Boards 1 2 and 3/4.3.3.1.2 controller basic cycle 0.2/Send can message5/CAN send ==
  In1 : Inport
  In2 : Inport  Port=2
  Gnd{3..9} (7 alike) : Ground
  S-Function : M-S-Function  FunctionName=sfcn_can_send  Parameters=tsamp, canBus, frameType, inputNumber, dataType, byteOrder
  wires:
  In1/1 -> S-Function/1
  In2/1 -> S-Function/2
  Gnd3/1 -> S-Function/3
  Gnd4/1 -> S-Function/4
  Gnd5/1 -> S-Function/5
  Gnd6/1 -> S-Function/6
  Gnd7/1 -> S-Function/7
  Gnd8/1 -> S-Function/8
  Gnd9/1 -> S-Function/9

== system HANcoder_E407_DYS_MP/HANcoder STM32 Target - E407-STM32 algorithm/4.TTA Can System/4.3 TTA System/4.3.3 Matrix Cycle Manager/4.3.3.1 Controller Matrix Cycle Truck Boards 1 2 and 3/4.3.3.1.2 controller basic cycle 0.2/Send can message5/CAN send1 ==
  In1 : Inport
  In2 : Inport  Port=2
  Gnd{3..9} (7 alike) : Ground
  S-Function : M-S-Function  FunctionName=sfcn_can_send  Parameters=tsamp, canBus, frameType, inputNumber, dataType, byteOrder
  wires:
  In1/1 -> S-Function/1
  In2/1 -> S-Function/2
  Gnd3/1 -> S-Function/3
  Gnd4/1 -> S-Function/4
  Gnd5/1 -> S-Function/5
  Gnd6/1 -> S-Function/6
  Gnd7/1 -> S-Function/7
  Gnd8/1 -> S-Function/8
  Gnd9/1 -> S-Function/9

== system HANcoder_E407_DYS_MP/HANcoder STM32 Target - E407-STM32 algorithm/4.TTA Can System/4.3 TTA System/4.3.3 Matrix Cycle Manager/4.3.3.1 Controller Matrix Cycle Truck Boards 1 2 and 3/4.3.3.1.2 controller basic cycle 0.2/Send can message6/CAN send ==
  In1 : Inport
  In2 : Inport  Port=2
  Gnd{3..9} (7 alike) : Ground
  S-Function : M-S-Function  FunctionName=sfcn_can_send  Parameters=tsamp, canBus, frameType, inputNumber, dataType, byteOrder
  wires:
  In1/1 -> S-Function/1
  In2/1 -> S-Function/2
  Gnd3/1 -> S-Function/3
  Gnd4/1 -> S-Function/4
  Gnd5/1 -> S-Function/5
  Gnd6/1 -> S-Function/6
  Gnd7/1 -> S-Function/7
  Gnd8/1 -> S-Function/8
  Gnd9/1 -> S-Function/9

== system HANcoder_E407_DYS_MP/HANcoder STM32 Target - E407-STM32 algorithm/4.TTA Can System/4.3 TTA System/4.3.3 Matrix Cycle Manager/4.3.3.1 Controller Matrix Cycle Truck Boards 1 2 and 3/4.3.3.1.2 controller basic cycle 0.2/Send can message6/CAN send1 ==
  In1 : Inport
  In2 : Inport  Port=2
  Gnd{3..9} (7 alike) : Ground
  S-Function : M-S-Function  FunctionName=sfcn_can_send  Parameters=tsamp, canBus, frameType, inputNumber, dataType, byteOrder
  wires:
  In1/1 -> S-Function/1
  In2/1 -> S-Function/2
  Gnd3/1 -> S-Function/3
  Gnd4/1 -> S-Function/4
  Gnd5/1 -> S-Function/5
  Gnd6/1 -> S-Function/6
  Gnd7/1 -> S-Function/7
  Gnd8/1 -> S-Function/8
  Gnd9/1 -> S-Function/9

== system HANcoder_E407_DYS_MP/HANcoder STM32 Target - E407-STM32 algorithm/4.TTA Can System/4.3 TTA System/4.3.3 Matrix Cycle Manager/4.3.3.1 Controller Matrix Cycle Truck Boards 1 2 and 3/4.3.3.1.2 controller basic cycle 0.2/Send can message7/CAN send ==
  In1 : Inport
  In2 : Inport  Port=2
  Gnd{3..9} (7 alike) : Ground
  S-Function : M-S-Function  FunctionName=sfcn_can_send  Parameters=tsamp, canBus, frameType, inputNumber, dataType, byteOrder
  wires:
  In1/1 -> S-Function/1
  In2/1 -> S-Function/2
  Gnd3/1 -> S-Function/3
  Gnd4/1 -> S-Function/4
  Gnd5/1 -> S-Function/5
  Gnd6/1 -> S-Function/6
  Gnd7/1 -> S-Function/7
  Gnd8/1 -> S-Function/8
  Gnd9/1 -> S-Function/9

== system HANcoder_E407_DYS_MP/HANcoder STM32 Target - E407-STM32 algorithm/4.TTA Can System/4.3 TTA System/4.3.3 Matrix Cycle Manager/4.3.3.1 Controller Matrix Cycle Truck Boards 1 2 and 3/4.3.3.1.2 controller basic cycle 0.2/Send can message7/CAN send1 ==
  In1 : Inport
  In2 : Inport  Port=2
  Gnd{3..9} (7 alike) : Ground
  S-Function : M-S-Function  FunctionName=sfcn_can_send  Parameters=tsamp, canBus, frameType, inputNumber, dataType, byteOrder
  wires:
  In1/1 -> S-Function/1
  In2/1 -> S-Function/2
  Gnd3/1 -> S-Function/3
  Gnd4/1 -> S-Function/4
  Gnd5/1 -> S-Function/5
  Gnd6/1 -> S-Function/6
  Gnd7/1 -> S-Function/7
  Gnd8/1 -> S-Function/8
  Gnd9/1 -> S-Function/9

== system HANcoder_E407_DYS_MP/HANcoder STM32 Target - E407-STM32 algorithm/4.TTA Can System/4.3 TTA System/4.3.3 Matrix Cycle Manager/4.3.3.2 Controller Matrix Cycle_Board 4 and 5/controller basic cycle 0/Receive Timer can master message /Receive can message ==
  Can_ID : Inport
  Enable : EnablePort  ShowOutputPort=on
  CAN receive : Subsystem  Tag=HANcoder_TARGET_STM32_E407  AncestorBlock=HANcoder_STM32_Target/STM32-E407/CAN/CAN/CAN receive  mask(CAN receive){canBus=CAN 1, outputNumber=1, dataType=uint8, byteOrder=off, tsamp=-1}
      mask prompts: canBus "CAN channel"; outputNumber "Output ports"; dataType "Output datatype"; byteOrder "Byte order: Checked = MSB first, unchecked = LSB first."; tsamp "Sample time"
      mask help:
      | Function
      | ==========
      | Receive the newest message from the specified CAN channel.
      |
      | Parameters
      | ==========
      | CAN channel:             The CAN channel to send the message on.
      | Output ports:             The amount of output ports
      | Output datatype:       The datatype of the output ports
      | Byte order:                 Select MSB or LSB first
      | Sample time:              -1 or divisible by base sample time [seconds]
      |
      | Input
      | ==========
      | Port 1:                       CAN ID(uint32) in hexadecimal ie: hex2dec('0a')
      |
      | Output
      | ==========
      | Port 1:                       Checks for new message(int8)
      | Port 2..9                     Message data
      mask init:
      | sfcn_can_receive_mcb(canBus, outputNumber, dataType, byteOrder)
      settings: MoveFcn=drawLogos
      mask Help: web('sfcn_can_receive.html');
      mask TypeOptions canBus: CAN 1 | CAN 2
      mask TypeOptions dataType: int8 | uint8 | int16 | uint16 | int32 | uint32 | boolean
      mask Display:
      | fprintf('Receive on\nCAN %x', canBus);
      | port_label('output', 1, 'new');
      | port_label('input', 1, 'ID');patch([75 81 81],[8 14 2],[1 0 0]);patch([83 83 89],[14 2 8],[0 0 0.35]);
  CAN receive2 : Subsystem  Tag=HANcoder_TARGET_STM32_E407  AncestorBlock=HANcoder_STM32_Target/STM32-E407/CAN/CAN/CAN receive  mask(CAN receive){canBus=CAN 2, outputNumber=1, dataType=uint8, byteOrder=off, tsamp=-1}
      mask prompts: canBus "CAN channel"; outputNumber "Output ports"; dataType "Output datatype"; byteOrder "Byte order: Checked = MSB first, unchecked = LSB first."; tsamp "Sample time"
      mask help:
      | Function
      | ==========
      | Receive the newest message from the specified CAN channel.
      |
      | Parameters
      | ==========
      | CAN channel:             The CAN channel to send the message on.
      | Output ports:             The amount of output ports
      | Output datatype:       The datatype of the output ports
      | Byte order:                 Select MSB or LSB first
      | Sample time:              -1 or divisible by base sample time [seconds]
      |
      | Input
      | ==========
      | Port 1:                       CAN ID(uint32) in hexadecimal ie: hex2dec('0a')
      |
      | Output
      | ==========
      | Port 1:                       Checks for new message(int8)
      | Port 2..9                     Message data
      mask init:
      | sfcn_can_receive_mcb(canBus, outputNumber, dataType, byteOrder)
      settings: MoveFcn=drawLogos
      mask Help: web('sfcn_can_receive.html');
      mask TypeOptions canBus: CAN 1 | CAN 2
      mask TypeOptions dataType: int8 | uint8 | int16 | uint16 | int32 | uint32 | boolean
      mask Display:
      | fprintf('Receive on\nCAN %x', canBus);
      | port_label('output', 1, 'new');
      | port_label('input', 1, 'ID');patch([75 81 81],[8 14 2],[1 0 0]);patch([83 83 89],[14 2 8],[0 0 0.35]);
  Can1Port1 : Outport
  Can1Receive : Outport  Port=2
  Can2Port2 : Outport  Port=3
  Can2Receive : Outport  Port=4
  wires:
  CAN receive/2(Out2) -> Can1Port1/1
  CAN receive/1(Out1) -> Can1Receive/1
  Can_ID/1 -> CAN receive2/1(In1), CAN receive/1(In1)
  CAN receive2/1(Out1) -> Can2Receive/1
  CAN receive2/2(Out2) -> Can2Port2/1

== system HANcoder_E407_DYS_MP/HANcoder STM32 Target - E407-STM32 algorithm/4.TTA Can System/4.3 TTA System/4.3.3 Matrix Cycle Manager/4.3.3.2 Controller Matrix Cycle_Board 4 and 5/controller basic cycle 0.2/If Action Subsystem2/If Action Subsystem2 ==
  Enable : EnablePort  ShowOutputPort=on
  Data Store Read : DataStoreRead  DataStoreName=ValitdatedSteeringAngle
  Data Store Write : DataStoreWrite  DataStoreName=PWMValue
  wires:
  Data Store Read/1 -> Data Store Write/1

== system HANcoder_E407_DYS_MP/HANcoder STM32 Target - E407-STM32 algorithm/4.TTA Can System/4.3 TTA System/4.3.3 Matrix Cycle Manager/4.3.3.2 Controller Matrix Cycle_Board 4 and 5/controller basic cycle 0.2/Receive Trailer 1 board 4 input angel/Desync calculation ==
  New_msg_CAN1 : Inport
  Can1_Msg : Inport  Port=2
  Can2_Msg : Inport  Port=3
  Enable : EnablePort  ShowOutputPort=on
  Switch1 : Switch  Priority=22  Criteria=u2 > Threshold
  Vote : Outport
  wires:
  New_msg_CAN1/1 -> Switch1/2
  Can1_Msg/1 -> Switch1/1
  Can2_Msg/1 -> Switch1/3
  Switch1/1 -> Vote/1

== system HANcoder_E407_DYS_MP/HANcoder STM32 Target - E407-STM32 algorithm/4.TTA Can System/4.3 TTA System/4.3.3 Matrix Cycle Manager/4.3.3.2 Controller Matrix Cycle_Board 4 and 5/controller basic cycle 0.2/Receive Trailer 1 board 4 input angel/Receive can message ==
  Can_ID : Inport
  Enable : EnablePort  ShowOutputPort=on
  CAN receive : Subsystem  Tag=HANcoder_TARGET_STM32_E407  AncestorBlock=HANcoder_STM32_Target/STM32-E407/CAN/CAN/CAN receive  mask(CAN receive){canBus=CAN 1, outputNumber=1, dataType=uint8, byteOrder=off, tsamp=-1}
      mask prompts: canBus "CAN channel"; outputNumber "Output ports"; dataType "Output datatype"; byteOrder "Byte order: Checked = MSB first, unchecked = LSB first."; tsamp "Sample time"
      mask help:
      | Function
      | ==========
      | Receive the newest message from the specified CAN channel.
      |
      | Parameters
      | ==========
      | CAN channel:             The CAN channel to send the message on.
      | Output ports:             The amount of output ports
      | Output datatype:       The datatype of the output ports
      | Byte order:                 Select MSB or LSB first
      | Sample time:              -1 or divisible by base sample time [seconds]
      |
      | Input
      | ==========
      | Port 1:                       CAN ID(uint32) in hexadecimal ie: hex2dec('0a')
      |
      | Output
      | ==========
      | Port 1:                       Checks for new message(int8)
      | Port 2..9                     Message data
      mask init:
      | sfcn_can_receive_mcb(canBus, outputNumber, dataType, byteOrder)
      settings: MoveFcn=drawLogos
      mask Help: web('sfcn_can_receive.html');
      mask TypeOptions canBus: CAN 1 | CAN 2
      mask TypeOptions dataType: int8 | uint8 | int16 | uint16 | int32 | uint32 | boolean
      mask Display:
      | fprintf('Receive on\nCAN %x', canBus);
      | port_label('output', 1, 'new');
      | port_label('input', 1, 'ID');patch([75 81 81],[8 14 2],[1 0 0]);patch([83 83 89],[14 2 8],[0 0 0.35]);
  CAN receive2 : Subsystem  Tag=HANcoder_TARGET_STM32_E407  AncestorBlock=HANcoder_STM32_Target/STM32-E407/CAN/CAN/CAN receive  mask(CAN receive){canBus=CAN 2, outputNumber=1, dataType=uint8, byteOrder=off, tsamp=-1}
      mask prompts: canBus "CAN channel"; outputNumber "Output ports"; dataType "Output datatype"; byteOrder "Byte order: Checked = MSB first, unchecked = LSB first."; tsamp "Sample time"
      mask help:
      | Function
      | ==========
      | Receive the newest message from the specified CAN channel.
      |
      | Parameters
      | ==========
      | CAN channel:             The CAN channel to send the message on.
      | Output ports:             The amount of output ports
      | Output datatype:       The datatype of the output ports
      | Byte order:                 Select MSB or LSB first
      | Sample time:              -1 or divisible by base sample time [seconds]
      |
      | Input
      | ==========
      | Port 1:                       CAN ID(uint32) in hexadecimal ie: hex2dec('0a')
      |
      | Output
      | ==========
      | Port 1:                       Checks for new message(int8)
      | Port 2..9                     Message data
      mask init:
      | sfcn_can_receive_mcb(canBus, outputNumber, dataType, byteOrder)
      settings: MoveFcn=drawLogos
      mask Help: web('sfcn_can_receive.html');
      mask TypeOptions canBus: CAN 1 | CAN 2
      mask TypeOptions dataType: int8 | uint8 | int16 | uint16 | int32 | uint32 | boolean
      mask Display:
      | fprintf('Receive on\nCAN %x', canBus);
      | port_label('output', 1, 'new');
      | port_label('input', 1, 'ID');patch([75 81 81],[8 14 2],[1 0 0]);patch([83 83 89],[14 2 8],[0 0 0.35]);
  Can1Port1 : Outport
  Can1Receive : Outport  Port=2
  Can2Port2 : Outport  Port=3
  Can2Receive : Outport  Port=4
  wires:
  CAN receive/2(Out2) -> Can1Port1/1
  CAN receive/1(Out1) -> Can1Receive/1
  Can_ID/1 -> CAN receive2/1(In1), CAN receive/1(In1)
  CAN receive2/1(Out1) -> Can2Receive/1
  CAN receive2/2(Out2) -> Can2Port2/1

== system HANcoder_E407_DYS_MP/HANcoder STM32 Target - E407-STM32 algorithm/4.TTA Can System/4.3 TTA System/4.3.3 Matrix Cycle Manager/4.3.3.2 Controller Matrix Cycle_Board 4 and 5/controller basic cycle 0.2/Receive Trailer 2 board 5 input angel/Desync calculation ==
  New_msg_CAN1 : Inport
  Can1_Msg : Inport  Port=2
  Can2_Msg : Inport  Port=3
  Enable : EnablePort  ShowOutputPort=on
  Switch1 : Switch  Priority=22  Criteria=u2 > Threshold
  Vote : Outport
  wires:
  New_msg_CAN1/1 -> Switch1/2
  Can1_Msg/1 -> Switch1/1
  Can2_Msg/1 -> Switch1/3
  Switch1/1 -> Vote/1

== system HANcoder_E407_DYS_MP/HANcoder STM32 Target - E407-STM32 algorithm/4.TTA Can System/4.3 TTA System/4.3.3 Matrix Cycle Manager/4.3.3.2 Controller Matrix Cycle_Board 4 and 5/controller basic cycle 0.2/Receive Trailer 2 board 5 input angel/Receive can message ==
  Can_ID : Inport
  Enable : EnablePort  ShowOutputPort=on
  CAN receive : Subsystem  Tag=HANcoder_TARGET_STM32_E407  AncestorBlock=HANcoder_STM32_Target/STM32-E407/CAN/CAN/CAN receive  mask(CAN receive){canBus=CAN 1, outputNumber=1, dataType=uint8, byteOrder=off, tsamp=-1}
      mask prompts: canBus "CAN channel"; outputNumber "Output ports"; dataType "Output datatype"; byteOrder "Byte order: Checked = MSB first, unchecked = LSB first."; tsamp "Sample time"
      mask help:
      | Function
      | ==========
      | Receive the newest message from the specified CAN channel.
      |
      | Parameters
      | ==========
      | CAN channel:             The CAN channel to send the message on.
      | Output ports:             The amount of output ports
      | Output datatype:       The datatype of the output ports
      | Byte order:                 Select MSB or LSB first
      | Sample time:              -1 or divisible by base sample time [seconds]
      |
      | Input
      | ==========
      | Port 1:                       CAN ID(uint32) in hexadecimal ie: hex2dec('0a')
      |
      | Output
      | ==========
      | Port 1:                       Checks for new message(int8)
      | Port 2..9                     Message data
      mask init:
      | sfcn_can_receive_mcb(canBus, outputNumber, dataType, byteOrder)
      settings: MoveFcn=drawLogos
      mask Help: web('sfcn_can_receive.html');
      mask TypeOptions canBus: CAN 1 | CAN 2
      mask TypeOptions dataType: int8 | uint8 | int16 | uint16 | int32 | uint32 | boolean
      mask Display:
      | fprintf('Receive on\nCAN %x', canBus);
      | port_label('output', 1, 'new');
      | port_label('input', 1, 'ID');patch([75 81 81],[8 14 2],[1 0 0]);patch([83 83 89],[14 2 8],[0 0 0.35]);
  CAN receive2 : Subsystem  Tag=HANcoder_TARGET_STM32_E407  AncestorBlock=HANcoder_STM32_Target/STM32-E407/CAN/CAN/CAN receive  mask(CAN receive){canBus=CAN 2, outputNumber=1, dataType=uint8, byteOrder=off, tsamp=-1}
      mask prompts: canBus "CAN channel"; outputNumber "Output ports"; dataType "Output datatype"; byteOrder "Byte order: Checked = MSB first, unchecked = LSB first."; tsamp "Sample time"
      mask help:
      | Function
      | ==========
      | Receive the newest message from the specified CAN channel.
      |
      | Parameters
      | ==========
      | CAN channel:             The CAN channel to send the message on.
      | Output ports:             The amount of output ports
      | Output datatype:       The datatype of the output ports
      | Byte order:                 Select MSB or LSB first
      | Sample time:              -1 or divisible by base sample time [seconds]
      |
      | Input
      | ==========
      | Port 1:                       CAN ID(uint32) in hexadecimal ie: hex2dec('0a')
      |
      | Output
      | ==========
      | Port 1:                       Checks for new message(int8)
      | Port 2..9                     Message data
      mask init:
      | sfcn_can_receive_mcb(canBus, outputNumber, dataType, byteOrder)
      settings: MoveFcn=drawLogos
      mask Help: web('sfcn_can_receive.html');
      mask TypeOptions canBus: CAN 1 | CAN 2
      mask TypeOptions dataType: int8 | uint8 | int16 | uint16 | int32 | uint32 | boolean
      mask Display:
      | fprintf('Receive on\nCAN %x', canBus);
      | port_label('output', 1, 'new');
      | port_label('input', 1, 'ID');patch([75 81 81],[8 14 2],[1 0 0]);patch([83 83 89],[14 2 8],[0 0 0.35]);
  Can1Port1 : Outport
  Can1Receive : Outport  Port=2
  Can2Port2 : Outport  Port=3
  Can2Receive : Outport  Port=4
  wires:
  CAN receive/2(Out2) -> Can1Port1/1
  CAN receive/1(Out1) -> Can1Receive/1
  Can_ID/1 -> CAN receive2/1(In1), CAN receive/1(In1)
  CAN receive2/1(Out1) -> Can2Receive/1
  CAN receive2/2(Out2) -> Can2Port2/1

== system HANcoder_E407_DYS_MP/HANcoder STM32 Target - E407-STM32 algorithm/4.TTA Can System/4.3 TTA System/4.3.3 Matrix Cycle Manager/4.3.3.2 Controller Matrix Cycle_Board 4 and 5/controller basic cycle 0.2/Receive Truck 1 Board 1 Calc Steering Angle/Desync calculation ==
  New_msg_CAN1 : Inport
  Can1_Msg : Inport  Port=2
  Can2_Msg : Inport  Port=3
  Enable : EnablePort  ShowOutputPort=on
  Switch1 : Switch  Priority=22  Criteria=u2 > Threshold
  Vote : Outport
  wires:
  New_msg_CAN1/1 -> Switch1/2
  Can1_Msg/1 -> Switch1/1
  Can2_Msg/1 -> Switch1/3
  Switch1/1 -> Vote/1
